simulink model "Schema_a_blocchi_modello_termico"  (R2023b)
settings: Solver=VariableStepAuto  StartTime=0.0  StopTime=1000  RelTol=1e-3
values from neighbouring files (symbols this model uses):
  Cr = 0.1    [modello_termico.m]
  Cs = 100    [modello_termico.m]
  R1 = 0.1    [ciccio_ciccio.m]    (also in modello_termico.m = 1)
settings Model: Creator=simon  LastModifiedBy=simon

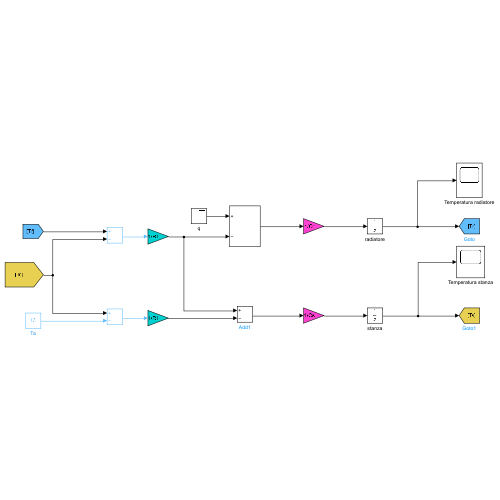
[thumbnail: Simulink's stored preview of the top-level diagram]
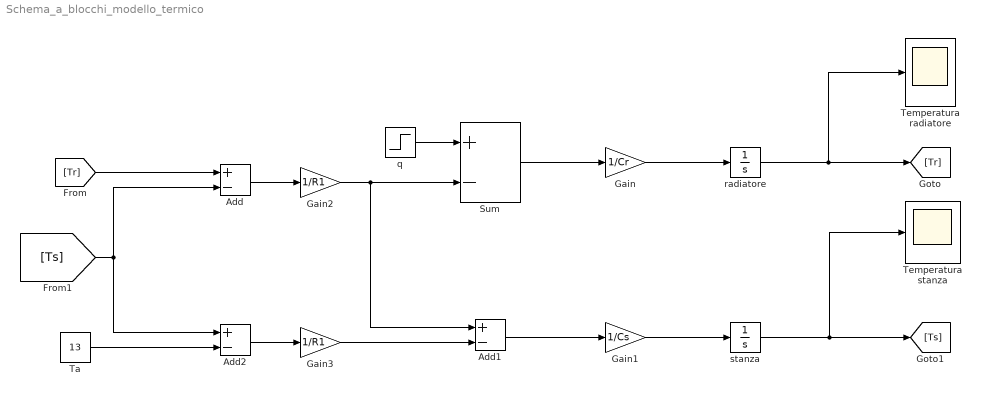
== system Schema_a_blocchi_modello_termico ==
  Add : Sum  Inputs=+-
  Add1 : Sum  Inputs=+-
  Add2 : Sum  Inputs=+-
  Gain : Gain  Gain=1/Cr
  Gain1 : Gain  Gain=1/Cs
  Gain2 : Gain  Gain=1/R1
  Gain3 : Gain  Gain=1/R1
  Sum : Sum  Inputs=+-
  Ta : Constant  Value=13
  Temperatura radiatore : Scope
  Temperatura stanza : Scope
  q : Step  Time=250  SampleTime=0
  radiatore : Integrator  InitialCondition=20
  stanza : Integrator  InitialCondition=8
  wires:
  Gain/1 -> radiatore/1
  Gain1/1 -> stanza/1
  Sum/1 -> Gain/1
  radiatore/1 -> Temperatura radiatore/1, [Tr]
  stanza/1 -> Temperatura stanza/1, [Ts]
  Gain2/1 -> Sum/2, Add1/1
  q/1 -> Sum/1
  [Tr] -> Add/1
  [Ts] -> Add/2, Add2/1
  Add/1 -> Gain2/1
  Ta/1 -> Add2/2
  Add2/1 -> Gain3/1
  Gain3/1 -> Add1/2
  Add1/1 -> Gain1/1
